simulink model "hw"  (R2022b)
settings: Solver=VariableStepAuto  StartTime=0.0  StopTime=10.0  RelTol=1e-3
values from neighbouring files (symbols this model uses):
  A2 = out.A2    [hw01.m]
  B1 = out.B1    [hw01.m]
  B2 = out.B2    [hw01.m]
  C2 = out.C2    [hw01.m]
settings Model: Creator=Wasif  LastModifiedBy=Wasif

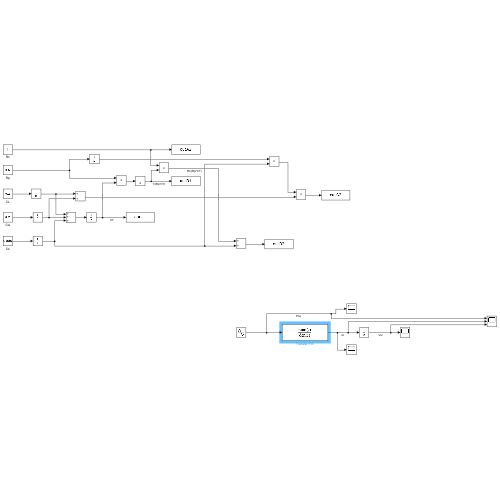
[thumbnail: Simulink's stored preview of the top-level diagram]
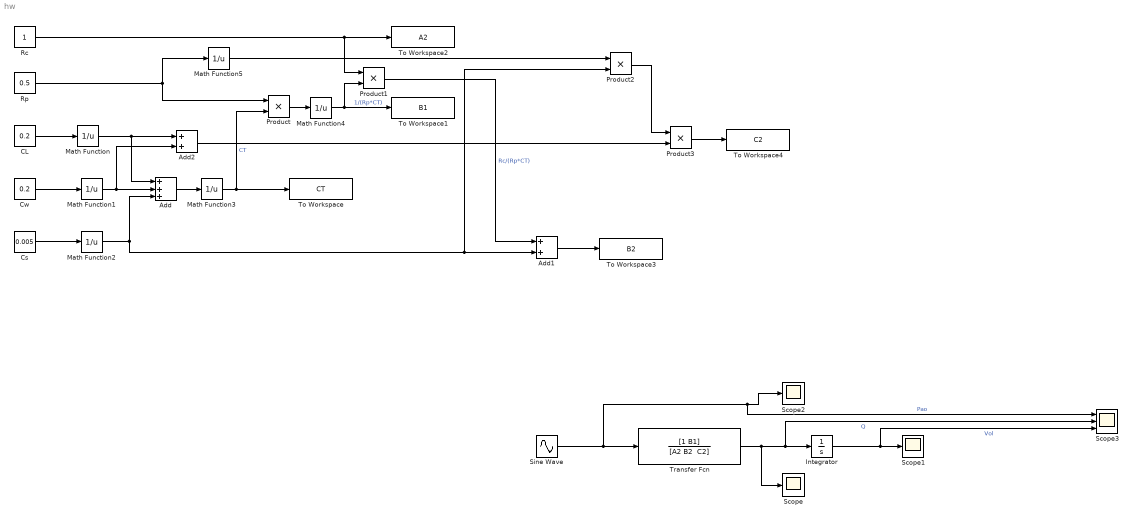
== system hw ==
  Add : Sum  Inputs=+++
  Add1 : Sum
  Add2 : Sum
  CL : Constant  Value=0.2
  Cs : Constant  Value=0.005
  Cw : Constant  Value=0.2
  Integrator : Integrator
  Math Function{,1..5} (6 alike) : Math  Operator=reciprocal
  Product{,1..3} (4 alike) : Product
  Rc : Constant
  Rp : Constant  Value=0.5
  Scope : Scope
  Scope1 : Scope
  Scope2 : Scope
  Scope3 : Scope  NumInputPorts=3
  Sine Wave : Sin  SampleTime=0
  To Workspace : ToWorkspace  VariableName=CT  SampleTime=-1
  To Workspace1 : ToWorkspace  VariableName=B1  SampleTime=-1
  To Workspace2 : ToWorkspace  VariableName=A2  SampleTime=-1
  To Workspace3 : ToWorkspace  VariableName=B2  SampleTime=-1
  To Workspace4 : ToWorkspace  VariableName=C2  SampleTime=-1
  Transfer Fcn : TransferFcn  Numerator=[1 B1]  Denominator="[A2 B2  C2]"
  wires:
  CL/1 -> Math Function/1
  Cw/1 -> Math Function1/1
  Cs/1 -> Math Function2/1
  Math Function/1 -> Add/1, Add2/1
  Math Function1/1 -> Add2/2, Add/2
  Math Function2/1 -> Add/3, Product2/2, Add1/2
  Math Function3/1 -> Product/2, To Workspace/1  "CT"
  Add/1 -> Math Function3/1
  Rp/1 -> Math Function5/1, Product/1
  Product/1 -> Math Function4/1
  Math Function4/1 -> Product1/2, To Workspace1/1  "1/(Rp*CT)"
  Rc/1 -> Product1/1, To Workspace2/1
  Product1/1 -> Add1/1  "Rc/(Rp*CT)"
  Add1/1 -> To Workspace3/1
  Math Function5/1 -> Product2/1
  Add2/1 -> Product3/2
  Product2/1 -> Product3/1
  Product3/1 -> To Workspace4/1
  Sine Wave/1 -> Scope3/1, Scope2/1, Transfer Fcn/1  "Pao"
  Transfer Fcn/1 -> Scope3/2, Integrator/1, Scope/1  "Q"
  Integrator/1 -> Scope3/3, Scope1/1  "Vol"
